simulink model "sincos"  (R2022a)
settings: Solver=FixedStepAuto  StartTime=0  StopTime=10  FixedStep=0.1  RelTol=1e-3
InitFcn:
  | Init_data
values from neighbouring files (symbols this model uses):
  dq0 = 0    [Init_data.m]
  dqm = [0,0,0,0].'    [Init_data.m]
  Kdbf = 5    [Init_data.m]
  Kdmf = diag([10,15,10,15])    [Init_data.m]
  Kibc = 1    [Init_data.m]
  Kibf = 1    [Init_data.m]
  Kimc = diag([1,1,1,1])    [Init_data.m]
  Kimf = diag([2,2,2,2])    [Init_data.m]
  Kpbc = 1    [Init_data.m]
  Kpbf = 10    [Init_data.m]
  Kpmc = diag([1,1,1,1])    [Init_data.m]
  Kpmf = diag([1,1,1,1])    [Init_data.m]
  q0 = 0.3    [Init_data.m]    (also in calc_Mass.m = w0)
  q0_d = 0    [Init_data.m]
  qm = [0.1,0.15,0.25,0.3].'    [Init_data.m]
  qm_d = [0,0,0,0].'    [Init_data.m]
settings Model: Creator=43840  LastModifiedBy=43840

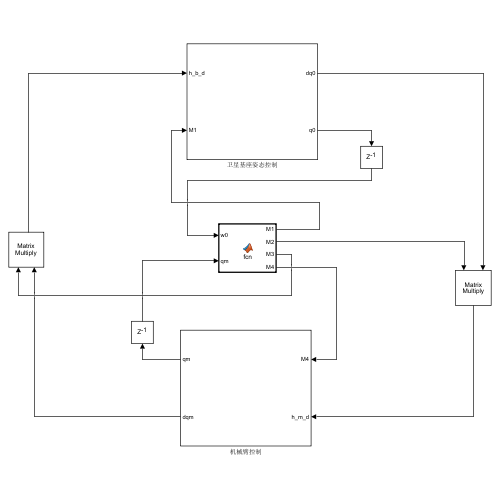
[thumbnail: Simulink's stored preview of the top-level diagram]
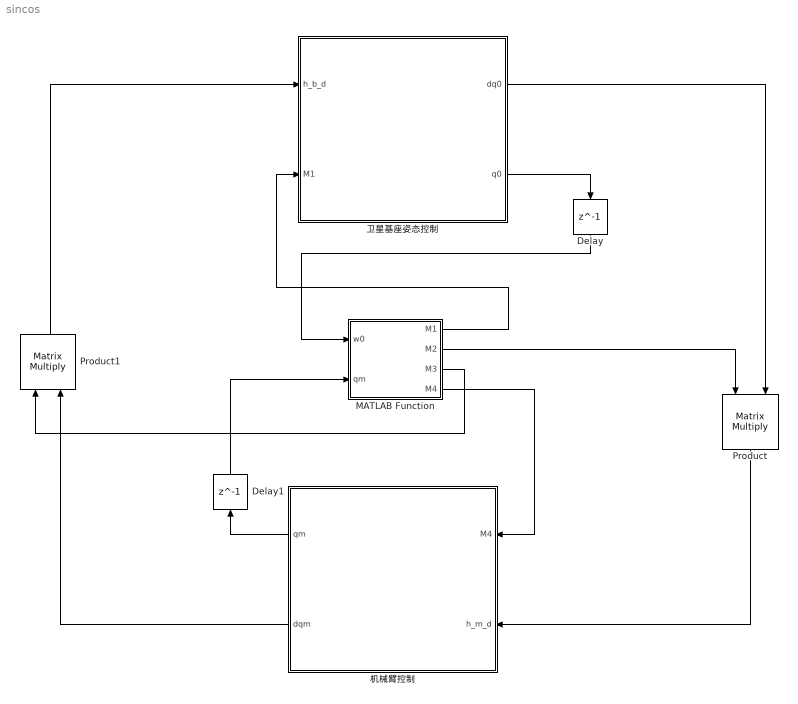
== system sincos ==
  Delay : Delay  DelayLength=1
  Delay1 : Delay  DelayLength=1
  MATLAB Function : MATLAB Function  TreatAsAtomicUnit=on
  Product : Product  Multiplication=Matrix(*)
  Product1 : Product  Multiplication=Matrix(*)
  卫星基座姿态控制 : Subsystem
  机械臂控制 : Subsystem
  wires:
  Product1/1 -> 卫星基座姿态控制/1(h_b_d)
  机械臂控制/2(dqm) -> Product1/2
  Product/1 -> 机械臂控制/2(h_m_d)
  卫星基座姿态控制/1(dq0) -> Product/2
  机械臂控制/1(qm) -> Delay1/1
  卫星基座姿态控制/2(q0) -> Delay/1
  MATLAB Function/1(M1) -> 卫星基座姿态控制/2(M1)
  MATLAB Function/4(M4) -> 机械臂控制/1(M4)
  MATLAB Function/2(M2) -> Product/1
  MATLAB Function/3(M3) -> Product1/1
  Delay/1 -> MATLAB Function/1(w0)
  Delay1/1 -> MATLAB Function/2(qm)

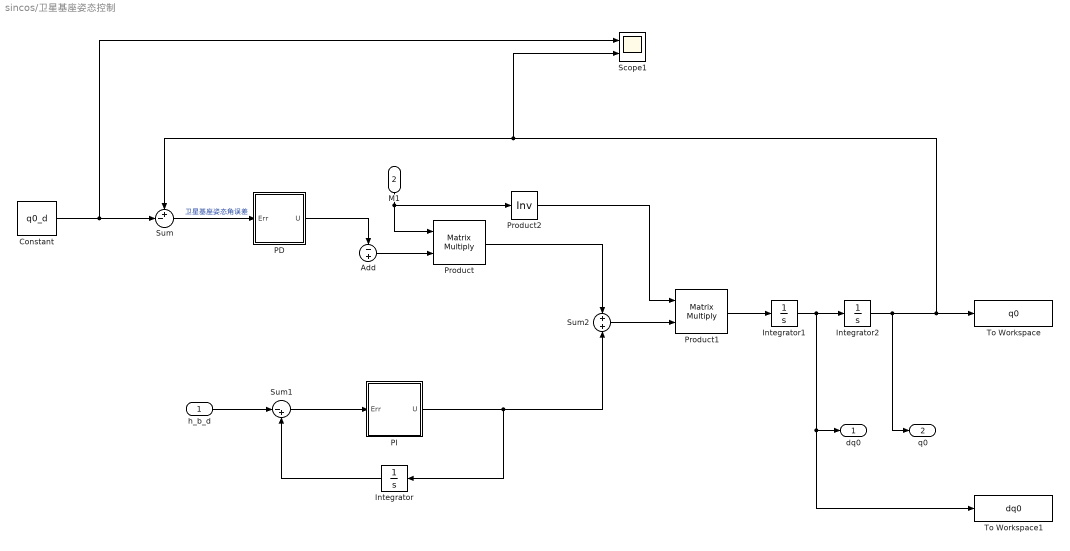
== system sincos/卫星基座姿态控制 ==
  h_b_d : Inport
  M1 : Inport  Port=2
  Add : Sum  Inputs=-+
  Constant : Constant  Value=q0_d  VectorParams1D=off
  Integrator : Integrator
  Integrator1 : Integrator  InitialCondition=dq0
  Integrator2 : Integrator  InitialCondition=q0
  PD : Subsystem
  PI : Subsystem
  Product : Product  Multiplication=Matrix(*)
  Product1 : Product  Multiplication=Matrix(*)
  Product2 : Product  Inputs=/  Multiplication=Matrix(*)
  Scope1 : Scope  NumInputPorts=2
  Sum : Sum  Inputs=+-|
  Sum1 : Sum  Inputs=|-+
  Sum2 : Sum  Inputs=+|+
  To Workspace : ToWorkspace  VariableName=q0  SampleTime=-1
      settings: Save2DSignal=2-D array (concatenate along first dimension)
  To Workspace1 : ToWorkspace  VariableName=dq0  SampleTime=-1
      settings: Save2DSignal=2-D array (concatenate along first dimension)
  dq0 : Outport
  q0 : Outport  Port=2
  wires:
  Sum/1 -> PD/1(Err)  "卫星基座姿态角误差"
  Integrator/1 -> Sum1/2
  Sum1/1 -> PI/1(Err)
  Product/1 -> Sum2/1
  PD/1(U) -> Add/1
  Add/1 -> Product/2
  PI/1(U) -> Sum2/2, Integrator/1
  h_b_d/1 -> Sum1/1
  Integrator1/1 -> Integrator2/1, To Workspace1/1, dq0/1
  Integrator2/1 -> q0/1, To Workspace/1, Scope1/2, Sum/1
  M1/1 -> Product2/1, Product/1
  Product2/1 -> Product1/1
  Product1/1 -> Integrator1/1
  Sum2/1 -> Product1/2
  Constant/1 -> Scope1/1, Sum/2

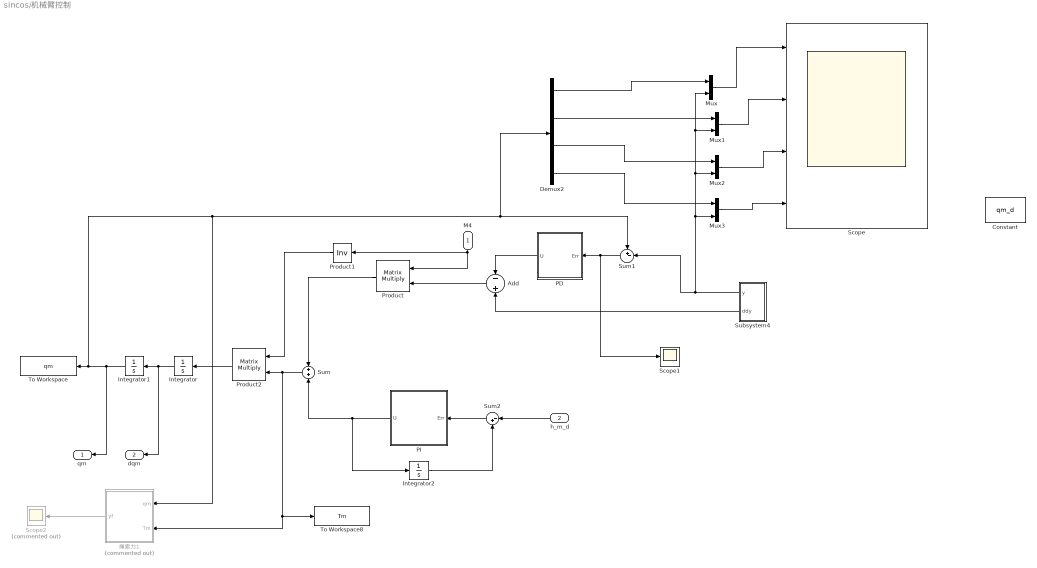
== system sincos/机械臂控制 ==
  M4 : Inport
  h_m_d : Inport  Port=2
  Add : Sum  Inputs=-+
  Constant : Constant  Value=qm_d
  Demux2 : Demux
  Integrator : Integrator  InitialCondition=dqm
  Integrator1 : Integrator  InitialCondition=qm
  Integrator2 : Integrator
  Mux{,1..3} (4 alike) : Mux  Inputs=2
  PD : Subsystem
  PI : Subsystem
  Product : Product  Multiplication=Matrix(*)
  Product1 : Product  Inputs=/  Multiplication=Matrix(*)
  Product2 : Product  Multiplication=Matrix(*)
  Scope : Scope  NumInputPorts=4
  Scope1 : Scope
  Scope2 : Scope  Commented=on
  Subsystem4 : Subsystem
  Sum : Sum
  Sum1 : Sum  Inputs=+-|
  Sum2 : Sum  Inputs=|-+
  To Workspace : ToWorkspace  VariableName=qm  SampleTime=-1
      settings: Save2DSignal=2-D array (concatenate along first dimension)
  To Workspace8 : ToWorkspace  VariableName=Tm  SampleTime=-1
      settings: Save2DSignal=2-D array (concatenate along first dimension)
  绳索力1 : MATLAB Function  Commented=on  TreatAsAtomicUnit=on
  qm : Outport
  dqm : Outport  Port=2
  wires:
  Integrator2/1 -> Sum2/2
  PI/1(U) -> Sum/2, Integrator2/1
  Sum2/1 -> PI/1(Err)
  Product2/1 -> Integrator/1
  Sum1/1 -> Scope1/1, PD/1(Err)
  Product/1 -> Sum/1
  Add/1 -> Product/2
  PD/1(U) -> Add/1
  h_m_d/1 -> Sum2/1
  M4/1 -> Product/1, Product1/1
  Integrator/1 -> dqm/1, Integrator1/1
  Product1/1 -> Product2/1
  Sum/1 -> 绳索力1/2(Tm), To Workspace8/1, Product2/2
  Integrator1/1 -> qm/1, To Workspace/1, Demux2/1, Sum1/1, 绳索力1/1(qm)
  Subsystem4/1(y) -> Mux2/2, Mux1/2, Mux/2, Mux3/2, Sum1/2
  Subsystem4/2(ddy) -> Add/2
  Mux2/1 -> Scope/3
  Mux/1 -> Scope/1
  Demux2/1 -> Mux/1
  Demux2/2 -> Mux1/1
  Mux1/1 -> Scope/2
  Demux2/3 -> Mux2/1
  Demux2/4 -> Mux3/1
  Mux3/1 -> Scope/4
  绳索力1/1(yf) -> Scope2/1

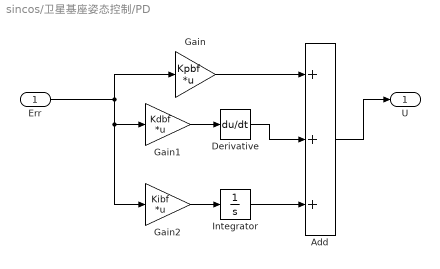
== system sincos/卫星基座姿态控制/PD ==
  Err : Inport
  Add : Sum  Inputs=+++
  Derivative : Derivative
  Gain : Gain  Gain=Kpbf  Multiplication=Matrix(K*u)
  Gain1 : Gain  Gain=Kdbf  Multiplication=Matrix(K*u)
  Gain2 : Gain  Gain=Kibf  Multiplication=Matrix(K*u)
  Integrator : Integrator
  U : Outport
  wires:
  Err/1 -> Gain2/1, Gain1/1, Gain/1
  Gain1/1 -> Derivative/1
  Gain/1 -> Add/1
  Derivative/1 -> Add/2
  Add/1 -> U/1
  Gain2/1 -> Integrator/1
  Integrator/1 -> Add/3

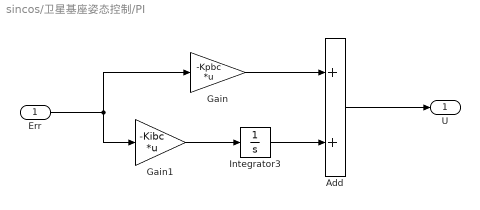
== system sincos/卫星基座姿态控制/PI ==
  Err : Inport
  Add : Sum
  Gain : Gain  Gain=-Kpbc  Multiplication=Matrix(K*u)
  Gain1 : Gain  Gain=-Kibc  Multiplication=Matrix(K*u)
  Integrator3 : Integrator
  U : Outport
  wires:
  Gain1/1 -> Integrator3/1
  Add/1 -> U/1
  Gain/1 -> Add/1
  Err/1 -> Gain1/1, Gain/1
  Integrator3/1 -> Add/2

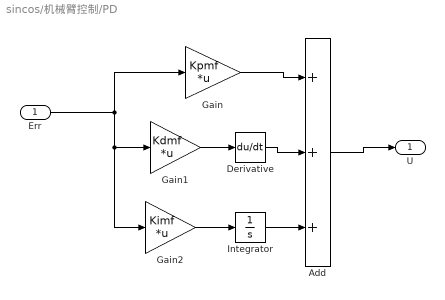
== system sincos/机械臂控制/PD ==
  Err : Inport
  Add : Sum  Inputs=+++
  Derivative : Derivative
  Gain : Gain  Gain=Kpmf  Multiplication=Matrix(K*u)
  Gain1 : Gain  Gain=Kdmf  Multiplication=Matrix(K*u)
  Gain2 : Gain  Gain=Kimf  Multiplication=Matrix(K*u)
  Integrator : Integrator
  U : Outport
  wires:
  Err/1 -> Gain2/1, Gain1/1, Gain/1
  Gain1/1 -> Derivative/1
  Gain/1 -> Add/1
  Derivative/1 -> Add/2
  Add/1 -> U/1
  Gain2/1 -> Integrator/1
  Integrator/1 -> Add/3

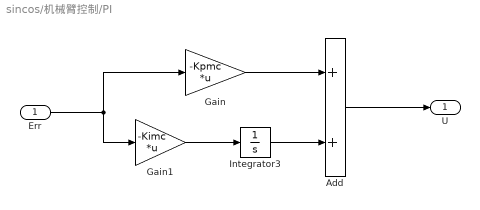
== system sincos/机械臂控制/PI ==
  Err : Inport
  Add : Sum
  Gain : Gain  Gain=-Kpmc  Multiplication=Matrix(K*u)
  Gain1 : Gain  Gain=-Kimc  Multiplication=Matrix(K*u)
  Integrator3 : Integrator
  U : Outport
  wires:
  Gain1/1 -> Integrator3/1
  Add/1 -> U/1
  Gain/1 -> Add/1
  Err/1 -> Gain1/1, Gain/1
  Integrator3/1 -> Add/2

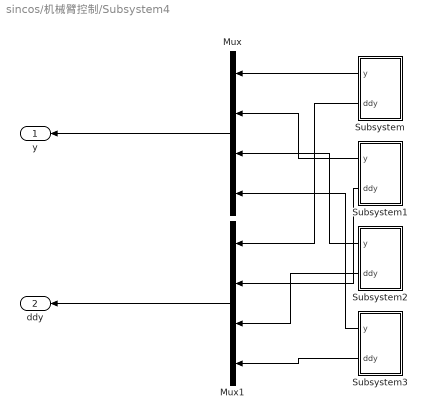
== system sincos/机械臂控制/Subsystem4 ==
  Mux : Mux
  Mux1 : Mux
  Subsystem : Subsystem
  Subsystem1 : Subsystem
  Subsystem2 : Subsystem
  Subsystem3 : Subsystem
  y : Outport
  ddy : Outport  Port=2
  wires:
  Subsystem1/2(ddy) -> Mux1/2
  Subsystem/2(ddy) -> Mux1/1
  Subsystem1/1(y) -> Mux/2
  Subsystem3/1(y) -> Mux/4
  Subsystem2/2(ddy) -> Mux1/3
  Subsystem2/1(y) -> Mux/3
  Subsystem3/2(ddy) -> Mux1/4
  Subsystem/1(y) -> Mux/1
  Mux/1 -> y/1
  Mux1/1 -> ddy/1

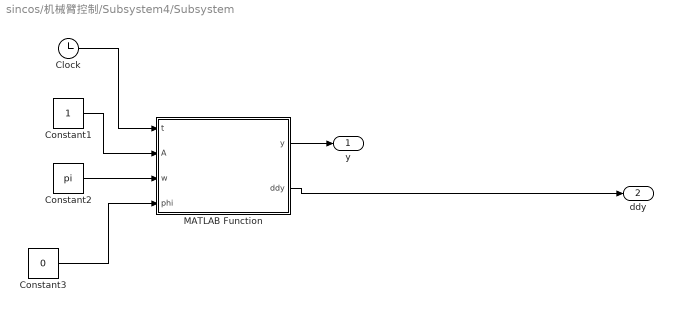
== system sincos/机械臂控制/Subsystem4/Subsystem ==
  Clock : Clock
  Constant1 : Constant
  Constant2 : Constant  Value=pi
  Constant3 : Constant  Value=0
  MATLAB Function : MATLAB Function  TreatAsAtomicUnit=on
  y : Outport
  ddy : Outport  Port=2
  wires:
  Clock/1 -> MATLAB Function/1(t)
  Constant1/1 -> MATLAB Function/2(A)
  MATLAB Function/2(ddy) -> ddy/1
  Constant3/1 -> MATLAB Function/4(phi)
  Constant2/1 -> MATLAB Function/3(w)
  MATLAB Function/1(y) -> y/1

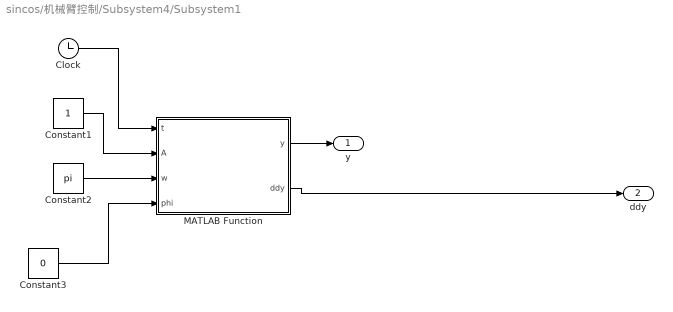
== system sincos/机械臂控制/Subsystem4/Subsystem1 ==
  Clock : Clock
  Constant1 : Constant
  Constant2 : Constant  Value=pi
  Constant3 : Constant  Value=0
  MATLAB Function : MATLAB Function  TreatAsAtomicUnit=on
  y : Outport
  ddy : Outport  Port=2
  wires:
  MATLAB Function/1(y) -> y/1
  Constant2/1 -> MATLAB Function/3(w)
  Constant3/1 -> MATLAB Function/4(phi)
  MATLAB Function/2(ddy) -> ddy/1
  Constant1/1 -> MATLAB Function/2(A)
  Clock/1 -> MATLAB Function/1(t)

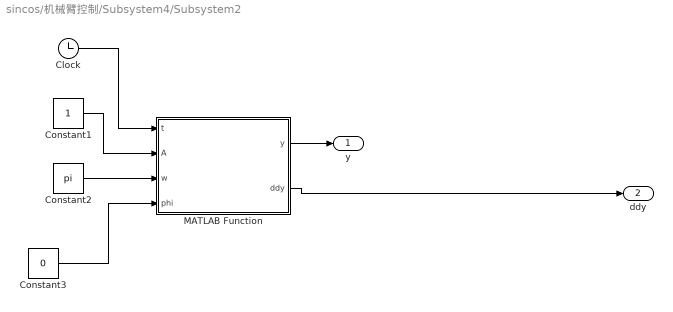
== system sincos/机械臂控制/Subsystem4/Subsystem2 ==
  Clock : Clock
  Constant1 : Constant
  Constant2 : Constant  Value=pi
  Constant3 : Constant  Value=0
  MATLAB Function : MATLAB Function  TreatAsAtomicUnit=on
  y : Outport
  ddy : Outport  Port=2
  wires:
  Clock/1 -> MATLAB Function/1(t)
  Constant1/1 -> MATLAB Function/2(A)
  MATLAB Function/2(ddy) -> ddy/1
  Constant3/1 -> MATLAB Function/4(phi)
  Constant2/1 -> MATLAB Function/3(w)
  MATLAB Function/1(y) -> y/1

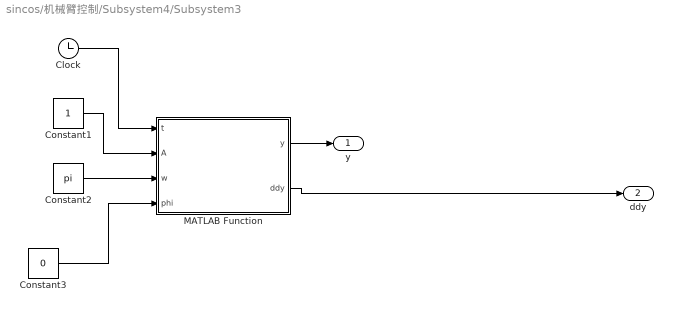
== system sincos/机械臂控制/Subsystem4/Subsystem3 ==
  Clock : Clock
  Constant1 : Constant
  Constant2 : Constant  Value=pi
  Constant3 : Constant  Value=0
  MATLAB Function : MATLAB Function  TreatAsAtomicUnit=on
  y : Outport
  ddy : Outport  Port=2
  wires:
  MATLAB Function/1(y) -> y/1
  Constant2/1 -> MATLAB Function/3(w)
  Constant3/1 -> MATLAB Function/4(phi)
  MATLAB Function/2(ddy) -> ddy/1
  Constant1/1 -> MATLAB Function/2(A)
  Clock/1 -> MATLAB Function/1(t)

== matlab function sincos/机械臂控制/Subsystem4/Subsystem/MATLAB Function ==
  data: t input; y output; A input; w input; phi input; ddy output
function [y,ddy] = fcn(t,A,w,phi)

y =A*sin(w*t+phi);
dy=A*w*sin(w*t+phi);
ddy=-A*w*w*sin(w*t+phi);

== matlab function sincos/MATLAB Function ==
  data: w0 input; M1 output; qm input; M2 output; M3 output; M4 output
function [M1, M2, M3, M4] = fcn(w0,qm)

coder.extrinsic("calc_Mass")

M1=zeros(1,1);
M2=zeros(4,1);
M3=zeros(1,4);
M4=zeros(4,4);

[M1, M2, M3, M4]=calc_Mass(w0,qm);

== matlab function sincos/机械臂控制/Subsystem4/Subsystem1/MATLAB Function ==
  data: t input; y output; A input; w input; phi input; ddy output
function [y,ddy] = fcn(t,A,w,phi)

y =A*sin(w*t+phi);
dy=A*w*sin(w*t+phi);
ddy=-A*w*w*sin(w*t+phi);

== matlab function sincos/机械臂控制/Subsystem4/Subsystem2/MATLAB Function ==
  data: t input; y output; A input; w input; phi input; ddy output
function [y,ddy] = fcn(t,A,w,phi)

y =A*sin(w*t+phi);
dy=A*w*sin(w*t+phi);
ddy=-A*w*w*sin(w*t+phi);

== matlab function sincos/机械臂控制/Subsystem4/Subsystem3/MATLAB Function ==
  data: t input; y output; A input; w input; phi input; ddy output
function [y,ddy] = fcn(t,A,w,phi)

y =A*sin(w*t+phi);
dy=A*w*sin(w*t+phi);
ddy=-A*w*w*sin(w*t+phi);

== matlab function sincos/机械臂控制/绳索力1 ==
  data: qm input; Tm input; yf output
function yf = fcn(qm,Tm)

coder.extrinsic("calc_J_hat")

yf=zeros(8,1);

yf=calc_J_hat(qm,Tm);
